simulink model "crc_8_general"  (R2021b)
settings: Solver=FixedStepDiscrete  StartTime=0.0  StopTime=0.01  FixedStep=0.01  RelTol=1e-3
libraries: msbUtilities x5, commcrc2 x1
settings Model: Creator=jekyll  LastModifiedBy=jekyll
settings OptimizationCC: DefaultParameterBehavior=Inlined  EnhancedBackFolding=on  PassReuseOutputArgsAs=Individual arguments  OptimizeBlockOrder=speed  DifferentSizesBufferReuse=on  OptimizationCustomize=off  EfficientTunableParamExpr=on
settings DebuggingCC: ParameterTunabilityLossMsg=error
settings SFSimCC: MATLABDynamicMemAlloc=off
settings RTWCC: Description=Embedded Coder  SystemTargetFile=ert.tlc  GenCodeOnly=on  TemplateMakefile=ert_default_tmf
settings CodeAppCC: ForceParamTrailComments=on  IgnoreCustomStorageClasses=off  OperatorAnnotations=on  SimulinkDataObjDesc=on  SFDataObjDesc=on  InsertBlockDesc=on
settings ERTTargetCC: TargetLangStandard=C99 (ISO)  GenerateSampleERTMain=on  SupportAbsoluteTime=off  CodeInterfacePackaging=Reusable function  SupportNonFinite=off  SupportComplex=off  InlinedParameterPlacement=NonHierarchical  ERTCustomFileTemplate=example_file_process.tlc

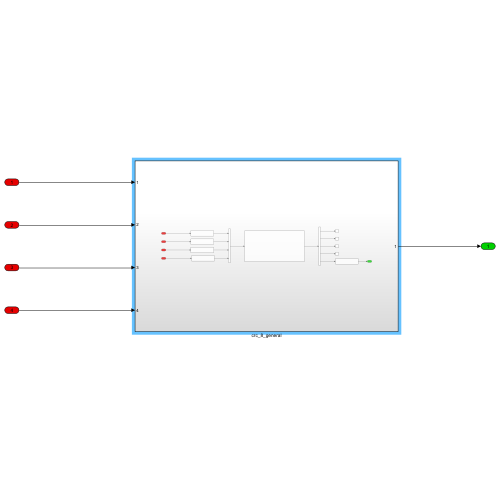
[thumbnail: Simulink's stored preview of the top-level diagram]
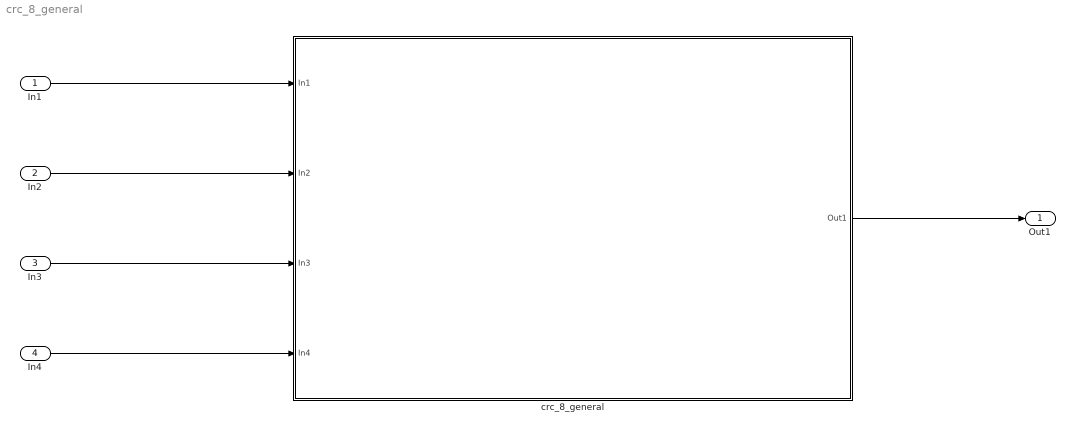
== system crc_8_general ==
  In1 : Inport  OutDataTypeStr=uint8
  In2 : Inport  Port=2  OutDataTypeStr=uint8
  In3 : Inport  Port=3  OutDataTypeStr=uint8
  In4 : Inport  Port=4  OutDataTypeStr=uint8
  crc_8_general : Subsystem
  Out1 : Outport  OutDataTypeStr=uint8
  wires:
  In2/1 -> crc_8_general/2(In2)
  crc_8_general/1(Out1) -> Out1/1
  In4/1 -> crc_8_general/4(In4)
  In1/1 -> crc_8_general/1(In1)
  In3/1 -> crc_8_general/3(In3)

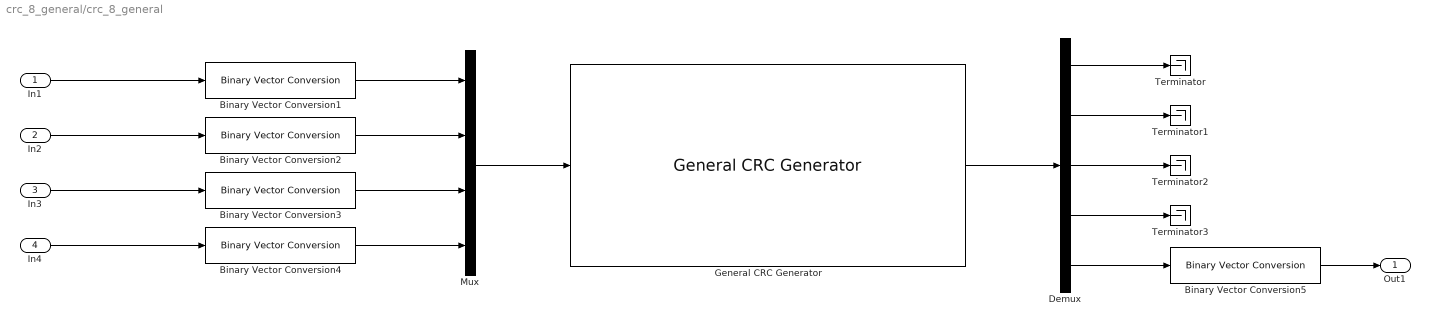
== system crc_8_general/crc_8_general ==
  In1 : Inport
  In2 : Inport  Port=2
  In3 : Inport  Port=3
  In4 : Inport  Port=4
  Binary Vector Conversion{1..4} (4 alike) : msbUtilities/Binary Vector Conversion  LabelModeActiveChoice=To Unipolar  Convert=Scalar to binary-coded vector  Encoding=Unipolar (magnitude)  InputLength=8  InputReverse=MSB at index 1  OutputLength=8  OutputReverse=MSB at index 1  DataType=uint8
      settings: SourceProductBaseCode=AM
  Binary Vector Conversion5 : msbUtilities/Binary Vector Conversion  LabelModeActiveChoice=From Unipolar  Convert=Binary-coded vector to scalar  Encoding=Unipolar (magnitude)  InputLength=8  InputReverse=MSB at index 1  OutputLength=8  OutputReverse=MSB at index 1  DataType=uint8
      settings: SourceProductBaseCode=AM
  Demux : Demux  Outputs=5
  General CRC Generator : commcrc2/General CRC Generator  genPoly='z^8 + z^4 + z^3 + z^2 + 1'  iniStates=1  directMethod=on  reflectInputBytes=off  reflectChecksums=off  finalXOR=1  numChecksums=1
      settings: SourceProductBaseCode=CM
  Mux : Mux
  Terminator{,1..3} (4 alike) : Terminator
  Out1 : Outport
  wires:
  Demux/2 -> Terminator1/1
  General CRC Generator/1 -> Demux/1
  Binary Vector Conversion3/1 -> Mux/3
  Mux/1 -> General CRC Generator/1
  In4/1 -> Binary Vector Conversion4/1
  Demux/3 -> Terminator2/1
  Binary Vector Conversion1/1 -> Mux/1
  In1/1 -> Binary Vector Conversion1/1
  Demux/1 -> Terminator/1
  Demux/5 -> Binary Vector Conversion5/1
  Binary Vector Conversion2/1 -> Mux/2
  In3/1 -> Binary Vector Conversion3/1
  In2/1 -> Binary Vector Conversion2/1
  Binary Vector Conversion4/1 -> Mux/4
  Demux/4 -> Terminator3/1
  Binary Vector Conversion5/1 -> Out1/1
